simulink model "movil_tray"  (R2015a)
settings: Solver=ode45  StartTime=0.0  StopTime=32  FixedStep=0.0001  RelTol=1e-3
undefined symbols (not defined in the file or in its folder): tipo_trayectoria
libraries: simulink x4
settings Model: Creator=Juan Esteban  LastModifiedBy=Juan Esteban

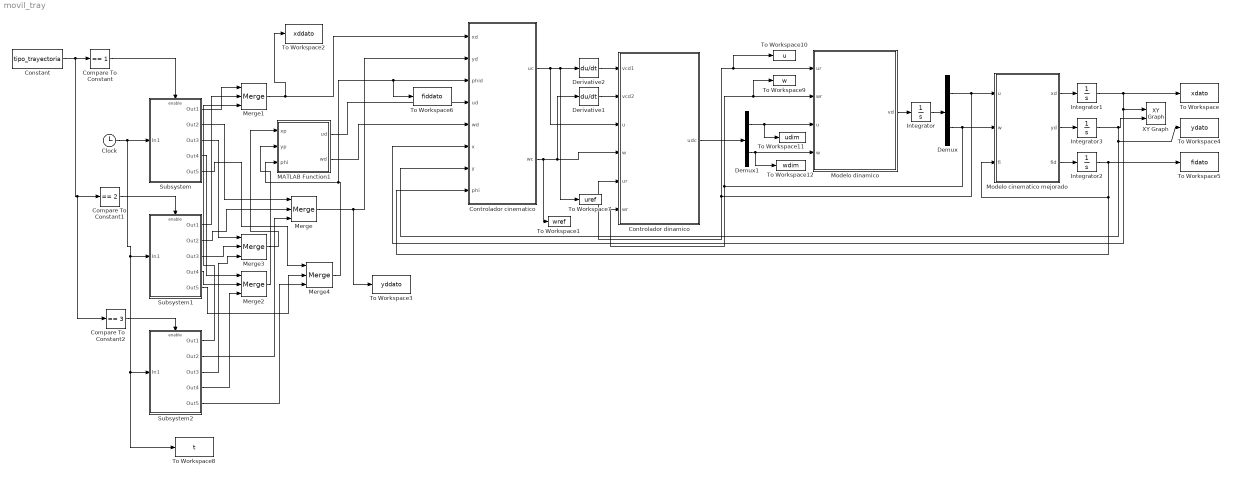
== system movil_tray ==
  Clock : Clock
  Compare To Constant : simulink/Logic and Bit Operations/Compare To Constant  relop===  const=1  OutDataTypeStr=boolean
  Compare To Constant1 : simulink/Logic and Bit Operations/Compare To Constant  relop===  const=2  OutDataTypeStr=boolean
  Compare To Constant2 : simulink/Logic and Bit Operations/Compare To Constant  relop===  const=3  OutDataTypeStr=boolean
  Constant : Constant  Value=tipo_trayectoria
  "Controlador cinematico " : MATLAB Function  TreatAsAtomicUnit=on
  Controlador dinamico : MATLAB Function  TreatAsAtomicUnit=on
  Demux : Demux  Outputs=2
  Demux1 : Demux  Outputs=2
  Derivative1 : Derivative
  Derivative2 : Derivative
  Integrator{,1..3} (4 alike) : Integrator
  MATLAB Function1 : MATLAB Function  TreatAsAtomicUnit=on
  Merge{,1..4} (5 alike) : Merge  Inputs=3
  Modelo cinematico mejorado : MATLAB Function  TreatAsAtomicUnit=on
  Modelo dinamico : MATLAB Function  TreatAsAtomicUnit=on
  Subsystem : Subsystem
  Subsystem1 : Subsystem
  Subsystem2 : Subsystem
  To Workspace : ToWorkspace  VariableName=xdato  SampleTime=-1
  To Workspace1 : ToWorkspace  VariableName=wref  SampleTime=-1
  To Workspace10 : ToWorkspace  VariableName=u  SampleTime=-1
  To Workspace11 : ToWorkspace  VariableName=udim  SampleTime=-1
  To Workspace12 : ToWorkspace  VariableName=wdim  SampleTime=-1
  To Workspace2 : ToWorkspace  VariableName=xddato  SampleTime=-1
  To Workspace3 : ToWorkspace  VariableName=yddato  SampleTime=-1
  To Workspace4 : ToWorkspace  VariableName=ydato  SampleTime=-1
  To Workspace5 : ToWorkspace  VariableName=fidato  SampleTime=-1
  To Workspace6 : ToWorkspace  VariableName=fiddato  SampleTime=-1
  To Workspace7 : ToWorkspace  VariableName=uref  SampleTime=-1
  To Workspace8 : ToWorkspace  VariableName=t  SampleTime=-1
  To Workspace9 : ToWorkspace  VariableName=w  SampleTime=-1
  XY Graph : simulink/Sinks/XY Graph  xmin=-10  xmax=10  ymin=-10  ymax=10  st=-1
  wires:
  MATLAB Function1/1(ud) -> "Controlador cinematico "/4(ud)
  MATLAB Function1/2(wd) -> "Controlador cinematico "/5(wd)
  Demux/1 -> Controlador dinamico/5(ur), To Workspace10/1, Modelo dinamico/1(ur), Modelo cinematico mejorado/1(u)
  Controlador dinamico/1(udc) -> Demux1/1
  Integrator/1 -> Demux/1
  Modelo cinematico mejorado/2(yd) -> Integrator3/1
  Modelo cinematico mejorado/1(xd) -> Integrator1/1
  Derivative1/1 -> Controlador dinamico/2(vcd2)
  Derivative2/1 -> Controlador dinamico/1(vcd1)
  Demux/2 -> To Workspace9/1, Modelo dinamico/2(wr), Controlador dinamico/6(wr), Modelo cinematico mejorado/2(w)
  Modelo dinamico/1(vd) -> Integrator/1
  Modelo cinematico mejorado/3(fid) -> Integrator2/1
  Demux1/1 -> Modelo dinamico/3(u), To Workspace11/1
  Demux1/2 -> Modelo dinamico/4(w), To Workspace12/1
  "Controlador cinematico "/2(wc) -> To Workspace1/1, Derivative1/1, Controlador dinamico/4(w)
  "Controlador cinematico "/1(uc) -> To Workspace7/1, Derivative2/1, Controlador dinamico/3(u)
  Integrator1/1 -> To Workspace/1, "Controlador cinematico "/6(x), XY Graph/1
  Integrator3/1 -> To Workspace4/1, "Controlador cinematico "/7(y), XY Graph/2
  Clock/1 -> Subsystem2/1(In1), To Workspace8/1, Subsystem1/1(In1), Subsystem/1(In1)
  Constant/1 -> Compare To Constant2/1, Compare To Constant1/1, Compare To Constant/1
  Compare To Constant/1 -> Subsystem/Enable
  Compare To Constant1/1 -> Subsystem1/Enable
  Subsystem/1(Out1) -> Merge1/1
  Subsystem1/1(Out1) -> Merge1/2
  Merge1/1 -> To Workspace2/1, "Controlador cinematico "/1(xd)
  Subsystem/2(Out2) -> Merge/1
  Subsystem1/2(Out2) -> Merge/2
  Merge/1 -> To Workspace3/1, "Controlador cinematico "/2(yd)
  Subsystem1/3(Out3) -> Merge3/2
  Subsystem/3(Out3) -> Merge3/1
  Merge3/1 -> MATLAB Function1/1(xp)
  Subsystem/4(Out4) -> Merge2/1
  Subsystem1/4(Out4) -> Merge2/2
  Merge2/1 -> MATLAB Function1/2(yp)
  Subsystem/5(Out5) -> Merge4/1
  Subsystem1/5(Out5) -> Merge4/2
  Merge4/1 -> To Workspace6/1, "Controlador cinematico "/3(phid), MATLAB Function1/3(phi)
  Integrator2/1 -> "Controlador cinematico "/8(phi), Modelo cinematico mejorado/3(fi), To Workspace5/1
  Compare To Constant2/1 -> Subsystem2/Enable
  Subsystem2/1(Out1) -> Merge1/3
  Subsystem2/3(Out3) -> Merge3/3
  Subsystem2/5(Out5) -> Merge4/3
  Subsystem2/2(Out2) -> Merge/3
  Subsystem2/4(Out4) -> Merge2/3

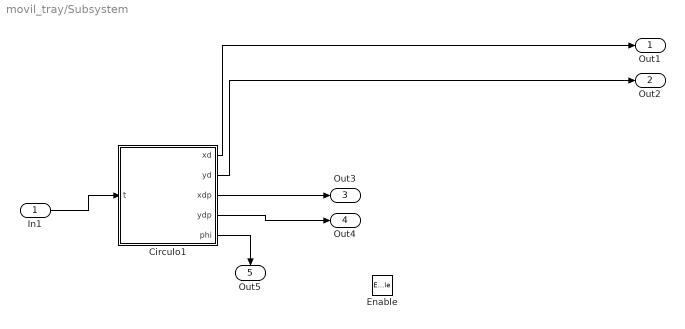
== system movil_tray/Subsystem ==
  In1 : Inport
  Enable : EnablePort
  Circulo1 : MATLAB Function  TreatAsAtomicUnit=on
  Out1 : Outport
  Out2 : Outport  Port=2
  Out3 : Outport  Port=3
  Out4 : Outport  Port=4
  Out5 : Outport  Port=5
  wires:
  In1/1 -> Circulo1/1(t)
  Circulo1/4(ydp) -> Out4/1
  Circulo1/5(phi) -> Out5/1
  Circulo1/3(xdp) -> Out3/1
  Circulo1/2(yd) -> Out2/1
  Circulo1/1(xd) -> Out1/1

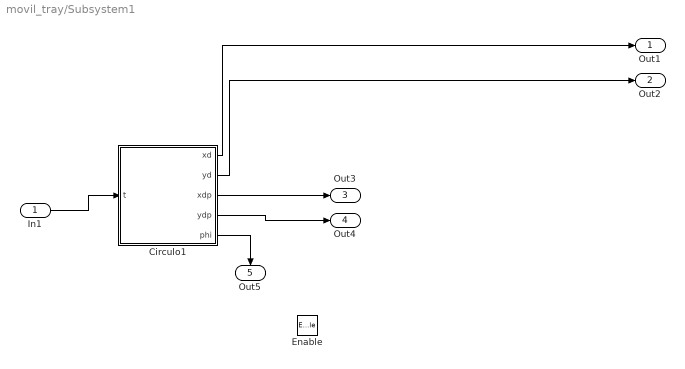
== system movil_tray/Subsystem1 ==
  In1 : Inport
  Enable : EnablePort
  Circulo1 : MATLAB Function  TreatAsAtomicUnit=on
  Out1 : Outport
  Out2 : Outport  Port=2
  Out3 : Outport  Port=3
  Out4 : Outport  Port=4
  Out5 : Outport  Port=5
  wires:
  In1/1 -> Circulo1/1(t)
  Circulo1/4(ydp) -> Out4/1
  Circulo1/5(phi) -> Out5/1
  Circulo1/3(xdp) -> Out3/1
  Circulo1/2(yd) -> Out2/1
  Circulo1/1(xd) -> Out1/1

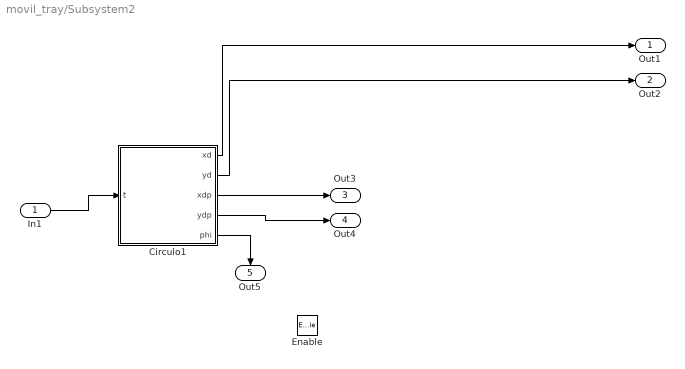
== system movil_tray/Subsystem2 ==
  In1 : Inport
  Enable : EnablePort
  Circulo1 : MATLAB Function  TreatAsAtomicUnit=on
  Out1 : Outport
  Out2 : Outport  Port=2
  Out3 : Outport  Port=3
  Out4 : Outport  Port=4
  Out5 : Outport  Port=5
  wires:
  In1/1 -> Circulo1/1(t)
  Circulo1/4(ydp) -> Out4/1
  Circulo1/5(phi) -> Out5/1
  Circulo1/3(xdp) -> Out3/1
  Circulo1/2(yd) -> Out2/1
  Circulo1/1(xd) -> Out1/1

== matlab function movil_tray/Modelo cinematico mejorado ==
  data: u input; w input; xd output; fi input; yd output; fid output
function [xd,yd,fid]= fcn(u,w,fi)
%#codegen
a=0.1;
xd=u*cos(fi)-a*w*sin(fi);
yd=u*sin(fi)-a*w*cos(fi);
fid=w;

== matlab function movil_tray/Controlador cinematico  ==
  data: xd input; yd input; phid input; ud input; wd input; x input; y input; phi input; uc output; wc output
function [uc,wc] = control(xd,yd,phid,ud,wd,x,y,phi)

e=[cos(phi) sin(phi) 0;-sin(phi) cos(phi) 0;0 0 1]*[xd-x;yd-y;phid-phi];
  e1=e(1);
  e2=e(2);
  e3=e(3);
  k1=4;
  k2=300;
  k3=200;
  mu1=-k1*e1;
  mu2=-k2*ud*(sin(e3)/e3)*e2-k3*e3;
  wc=wd-mu2;
  uc=ud*cos(e3)-mu1;

== matlab function movil_tray/Controlador dinamico ==
  data: vcd1 input; vcd2 input; u input; w input; ur input; wr input; udc output
function udc = fcn(vcd1,vcd2,u,w,ur,wr)
%#codegen
theta1=0.4072;
theta2=0.2937;
theta3=-0.0287;
theta4=0.9979;
theta5=-0.0004;
theta6=0.9865;
Qd=[2000 0;0 2000];
Kd=[100 0;0 100];
vcd=[vcd1;vcd2];
M=[theta1 0;0 theta2];
theta=[theta1 theta2 theta3 theta4 theta5 theta6]';
n=[0 0 -(wr^2) ur 0 0;0 0 0 0 wr*ur wr]*theta;
ve=[(u-ur);(w-wr)];
sigma=vcd+Qd*tanh(inv(Qd)*Kd*ve);
udc=M*sigma+n;

== matlab function movil_tray/Subsystem/Circulo1 ==
  data: xd output; yd output; xdp output; ydp output; phi output; t input
function [xd,yd,xdp,ydp,phi] = trayectoria(t)
yd=5*sin(t/5);
xd=5*cos(t/5);
ydp=5*cos(t/5)/5;
xdp=-5*sin(t/5)/5;
phi=atan2(ydp,xdp);

== matlab function movil_tray/Modelo dinamico ==
  data: ur input; wr input; u input; vd output; w input
function vd = fcn(ur,wr,u,w)
%#codegen
theta1=0.4072;
theta2=0.2937;
theta3=-0.0287;
theta4=0.9979;
theta5=-0.0004;
theta6=0.9865;
M=[theta1 0;0 theta2];
theta=[theta1 theta2 theta3 theta4 theta5 theta6]';
n=[0 0 -(wr^2) ur 0 0;0 0 0 0 wr*ur wr]*theta;
ud=[u;w];
vd=inv(M)*(ud-n);

== matlab function movil_tray/MATLAB Function1 ==
  data: ud output; xp input; yp input; phi input; wd output
function [ud,wd] = inversa(xp,yp,phi)
a=1;
J=[cos(phi) -a*sin(phi);...
    sin(phi) a*cos(phi)];
hp=[xp;yp];
vd=inv(J)*hp;
ud=vd(1);
wd=vd(2);

== matlab function movil_tray/Subsystem1/Circulo1 ==
  data: xd output; yd output; xdp output; ydp output; phi output; t input
function [xd,yd,xdp,ydp,phi] = trayectoria(t)
yd=5*sin(t/(5*0.5));
xd=5*cos(t/5);
ydp=5*cos(t/(5*0.5))/(5*0.5);
xdp=-5*sin(t/5)/5;
phi=atan2(ydp,xdp);

== matlab function movil_tray/Subsystem2/Circulo1 ==
  data: xd output; yd output; xdp output; ydp output; phi output; t input
function [xd,yd,xdp,ydp,phi] = trayectoria(t)
if t<=8
    yd=5;
    xd=1.25*t-5;
    xdp=1.25;
    ydp=0.001;
elseif t<=16
    xd=5;
    yd=-1.25*t+15;
    xdp=0.001;
    ydp=-1.25;
elseif t<=24
    yd=-5;
    xd=-1.25*t+25;
    ydp=0.001;
    xdp=-1.25;
elseif t<=32
    xd=-5;
    yd=1.25*t-35;
    xdp=0.001;
    ydp=1.25;
else
    xd=-5;
    yd=5;
    xdp=0.001;
    ydp=0.001;
end
phi=atan2(ydp,xdp);
